simulink subsystem "Motors"  (R2024b)
settings: Solver=VariableStepAuto  StartTime=0.0  StopTime=10.0  RelTol=1e-3
settings Model: Creator=JesseJabezArendse  LastModifiedBy=JesseJabezArendse
settings RTWCC: GPUComputeCapability=3.5

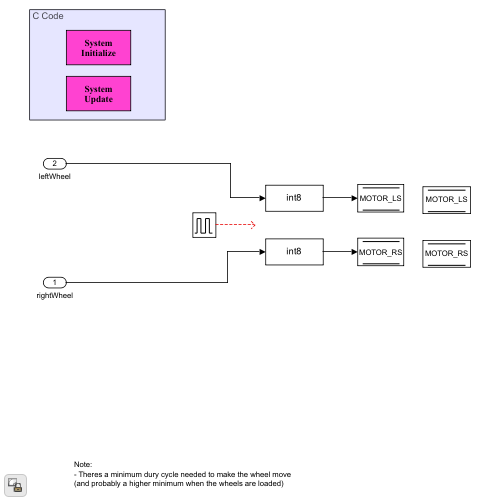
[thumbnail: Simulink's stored preview of the top-level diagram]
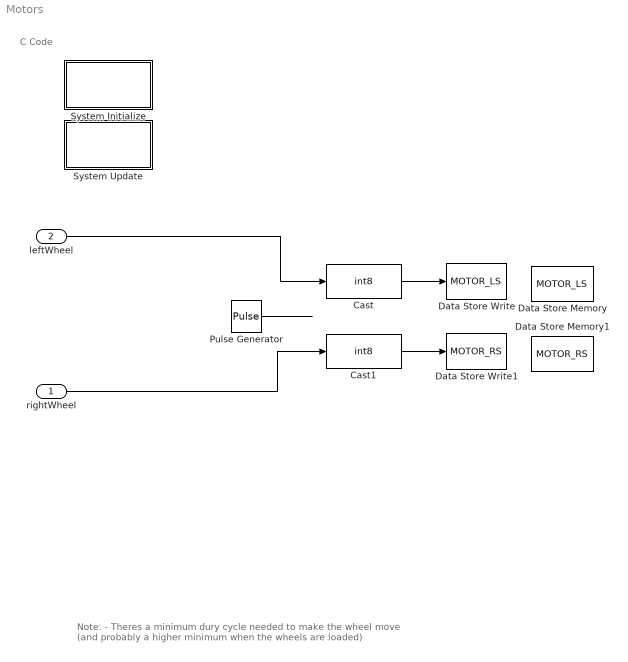
== system Motors ==
  note: Note:
      | - Theres a minimum dury cycle needed to make the wheel move (and probably a higher minimum when the wheels are loaded)
  note: C Code
  rightWheel : Inport  PortDimensions=1
  leftWheel : Inport  Port=2  PortDimensions=1
  Cast : DataTypeConversion  OutDataTypeStr=int8  SaturateOnIntegerOverflow=off  RndMeth=Floor
  Cast1 : DataTypeConversion  OutDataTypeStr=int8  SaturateOnIntegerOverflow=off  RndMeth=Floor
  Data Store Memory : DataStoreMemory  DataStoreName=MOTOR_LS  WriteAfterWriteMsg=warning  ShowAdditionalParam=off  OutDataTypeStr=int8  Dimensions=1
  Data Store Memory1 : DataStoreMemory  DataStoreName=MOTOR_RS  WriteAfterWriteMsg=warning  ShowAdditionalParam=off  OutDataTypeStr=int8  Dimensions=1
  Data Store Write : DataStoreWrite  DataStoreName=MOTOR_LS  IndexOptions=Index vector (dialog)  Indices=1  OutputSizes=1
  Data Store Write1 : DataStoreWrite  DataStoreName=MOTOR_RS  IndexOptions=Index vector (dialog)  Indices=1  OutputSizes=1
  Pulse Generator : DiscretePulseGenerator  PulseType=Time based  Period=0.04  PulseWidth=50
  System Initialize : Subsystem  mask(System Initialize){ShowInLibBrowser=0}
      mask prompts: ShowInLibBrowser "Simulink:masks:CustCodeMaskParam1_MP"
      settings: CopyFcn=cccopyfcn(gcb)  OpenFcn=ccopenfcn('System Initialize Function')
      mask Help: eval('feval(''rtwprivate'',''rtwhelpview'',''rtw_sys_initialize_block'')');
      mask Display: disp('System\nInitialize');
  System Update : Subsystem  mask(System Update){ShowInLibBrowser=0}
      mask prompts: ShowInLibBrowser "Simulink:masks:CustCodeMaskParam1_MP"
      settings: CopyFcn=cccopyfcn(gcb)  OpenFcn=ccopenfcn('System Update Function')
      mask Help: eval('feval(''rtwprivate'',''rtwhelpview'',''rtw_sys_update_block'')');
      mask Display: disp('System\nUpdate');
  wires:
  Pulse Generator/1 -> ?
  leftWheel/1 -> Cast/1
  rightWheel/1 -> Cast1/1
  Cast/1 -> Data Store Write/1
  Cast1/1 -> Data Store Write1/1

== system Motors/System Initialize ==

== system Motors/System Update ==
